simulink model "Simulink"  (R2021a)
settings: Solver=VariableStepAuto  StartTime=0.0  StopTime=10.0  RelTol=1e-3
settings Model: Creator=Santiago  LastModifiedBy=Santiago

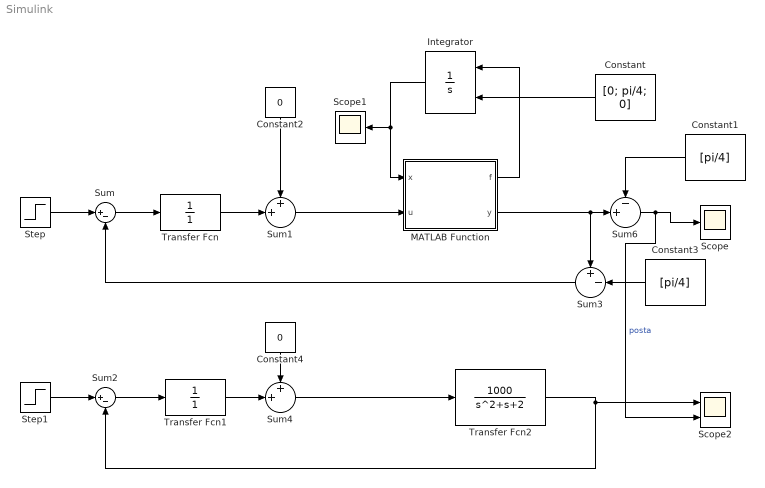
== system Simulink ==
  Constant : Constant  Value=[0; pi/4; 0]
  Constant1 : Constant  Value=[pi/4]
  Constant2 : Constant  Value=0
  Constant3 : Constant  Value=[pi/4]
  Constant4 : Constant  Value=0
  Integrator : Integrator  InitialConditionSource=external
  MATLAB Function : MATLAB Function  TreatAsAtomicUnit=on
  Scope : Scope
  Scope1 : Scope
  Scope2 : Scope  NumInputPorts=2
  Step : Step  After=0.2  SampleTime=0
  Step1 : Step  After=0.2  SampleTime=0
  Sum : Sum  Inputs=|+-
  Sum1 : Sum  Inputs=++|
  Sum2 : Sum  Inputs=|+-
  Sum3 : Sum  Inputs=+-|
  Sum4 : Sum  Inputs=++|
  Sum6 : Sum  Inputs=-+|
  Transfer Fcn : TransferFcn  Denominator=[1]
  Transfer Fcn1 : TransferFcn  Denominator=[1]
  Transfer Fcn2 : TransferFcn  Numerator=[1000]  Denominator=[1 1 2]
  wires:
  Step/1 -> Sum/1
  Sum/1 -> Transfer Fcn/1
  Sum1/1 -> MATLAB Function/2(u)
  MATLAB Function/1(f) -> Integrator/1
  Integrator/1 -> Scope1/1, MATLAB Function/1(x)
  Constant/1 -> Integrator/2
  Transfer Fcn/1 -> Sum1/2
  Constant2/1 -> Sum1/1
  Sum3/1 -> Sum/2
  Constant3/1 -> Sum3/2
  Step1/1 -> Sum2/1
  Constant4/1 -> Sum4/1
  Transfer Fcn1/1 -> Sum4/2
  Sum4/1 -> Transfer Fcn2/1
  Transfer Fcn2/1 -> Sum2/2, Scope2/1
  Sum2/1 -> Transfer Fcn1/1
  MATLAB Function/2(y) -> Sum3/1, Sum6/2
  Constant1/1 -> Sum6/1
  Sum6/1 -> Scope2/2, Scope/1  "posta"

== matlab function Simulink/MATLAB Function ==
  data: x input; f output; u input; y output
function [f, y] = fcn(x, u)

p = 1000;
alfa = (4/pi)^3 * 1/sqrt(2);;

f1 = -p * x(1) + p * u;
f2 = x(3);
f3 = -alfa * x(2)^3 + sin(x(2)) - x(3) + x(1);
f = [f1; f2; f3];

y = x(2);
